simulink model "soustava_diff_rovnic"  (R2021a)
settings: Solver=VariableStepAuto  StartTime=0.0  StopTime=20e-3  RelTol=1e-3
undefined symbols (not defined in the file): C, L, R1, R2, U_0
settings Model: Creator=vojte  LastModifiedBy=vojte

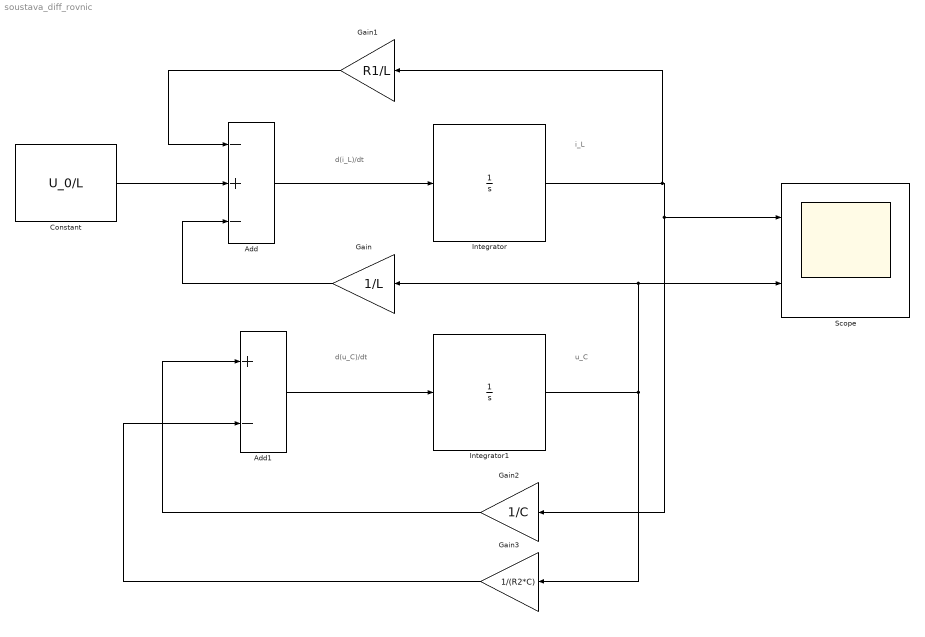
== system soustava_diff_rovnic ==
  note: i_L
  note: u_C
  note: d(u_C)/dt
  note: d(i_L)/dt
  Add : Sum  Inputs=-+-
  Add1 : Sum  Inputs=+-
  Constant : Constant  Value=U_0/L
  Gain : Gain  Gain=1/L
  Gain1 : Gain  Gain=R1/L
  Gain2 : Gain  Gain=1/C
  Gain3 : Gain  Gain=1/(R2*C)
  Integrator : Integrator
  Integrator1 : Integrator
  Scope : Scope  NumInputPorts=2
  wires:
  Add/1 -> Integrator/1
  Integrator1/1 -> Scope/2, Gain/1, Gain3/1
  Gain/1 -> Add/3
  Constant/1 -> Add/2
  Gain1/1 -> Add/1
  Gain2/1 -> Add1/1
  Gain3/1 -> Add1/2
  Add1/1 -> Integrator1/1
  Integrator/1 -> Gain1/1, Gain2/1, Scope/1
